simulink model "Surgical_RCM_Sim"  (R2026a)
settings: Solver=VariableStepAuto  StopTime=30.0
settings Model: Creator=shueb  LastModifiedBy=shueb

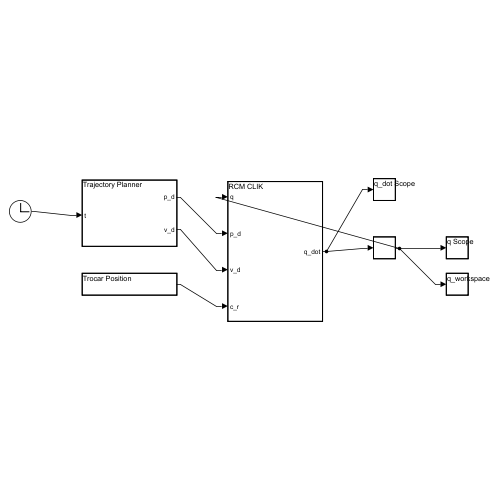
[thumbnail: Simulink's stored preview of the top-level diagram]
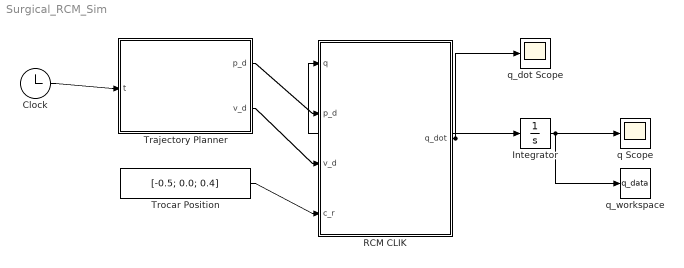
== system Surgical_RCM_Sim ==
  Clock : Clock
  Integrator : Integrator  InitialCondition=[0; 0.4085; 3.1416; 0.6128; -3.1416; 2.1203; 3.1416]
  RCM CLIK : MATLAB Function  TreatAsAtomicUnit=on
  Trajectory Planner : MATLAB Function  TreatAsAtomicUnit=on
  Trocar Position : Constant  Value=[-0.5; 0.0; 0.4]
  q Scope : Scope
  q_dot Scope : Scope
  q_workspace : ToWorkspace  VariableName=q_data  SampleTime=-1
  wires:
  Clock/1 -> Trajectory Planner/1(t)
  Trajectory Planner/1(p_d) -> RCM CLIK/2(p_d)
  Trajectory Planner/2(v_d) -> RCM CLIK/3(v_d)
  Trocar Position/1 -> RCM CLIK/4(c_r)
  Integrator/1 -> RCM CLIK/1(q), q Scope/1, q_workspace/1
  RCM CLIK/1(q_dot) -> Integrator/1, q_dot Scope/1

== matlab function Surgical_RCM_Sim/RCM CLIK ==
  data: q input; q_dot output; p_d input; v_d input; c_r input
function q_dot = rcm_clik_controller(q, p_d, v_d, c_r)
    %#codegen
    assert(isa(q, 'double'));
    assert(all(size(q) == [7, 1]));
    assert(isa(p_d, 'double'));
    assert(all(size(p_d) == [3, 1]));
    assert(isa(v_d, 'double'));
    assert(all(size(v_d) == [3, 1]));
    assert(isa(c_r, 'double'));
    assert(all(size(c_r) == [3, 1]));

    q_dot = zeros(7, 1);
    % Gains
    K_rcm = 10;
    K_tool = 5;
    
    % Forward Kinematics
    T_e = kuka_direct_kinematics(q);
    p_e = T_e(1:3, 4);
    R_e = T_e(1:3, 1:3);
    z_e = R_e(:, 3);
    
    J_e = jacobian_kuka(q);
    J_v = J_e(1:3, :);
    J_w = J_e(4:6, :);
    
    % Tool Kinematics
    L = 0.15;
    p_tool = p_e + L * z_e;
    skew_Lz = [0, -L*z_e(3), L*z_e(2);
               L*z_e(3), 0, -L*z_e(1);
               -L*z_e(2), L*z_e(1), 0];
    J_tool = J_v - skew_Lz * J_w;
    
    % RCM Kinematics
    lambda = (c_r - p_e)' * z_e;
    p_c = p_e + lambda * z_e;
    e_rcm = c_r - p_c;
    
    skew_lamz = [0, -lambda*z_e(3), lambda*z_e(2);
                 lambda*z_e(3), 0, -lambda*z_e(1);
                 -lambda*z_e(2), lambda*z_e(1), 0];
    J_pc = J_v - skew_lamz * J_w;
    
    Proj_ortho = eye(3) - z_e * z_e';
    J_rcm = Proj_ortho * J_pc;
    
    % Task-Priority CLIK
    % Task 1: RCM Constraint (highest priority)
    J_rcm_pinv = pinv(J_rcm);
    q_dot_1 = J_rcm_pinv * (K_rcm * e_rcm);
    
    % Task 2: Tool tracking (secondary priority)
    e_tool = p_d - p_tool;
    v_tool_1 = J_tool * q_dot_1;
    v_tool_req = v_d + K_tool * e_tool - v_tool_1;
    
    N_1 = eye(7) - J_rcm_pinv * J_rcm;
    J_tool_N = J_tool * N_1;
    
    % Damped Least Squares for Secondary Task to avoid singularities
    lambda_damp = 0.1;
    J_tool_N_pinv = J_tool_N' / (J_tool_N * J_tool_N' + lambda_damp^2 * eye(3));
    
    q_dot_2 = J_tool_N_pinv * v_tool_req;
    
    q_dot = q_dot_1 + q_dot_2;
end

== matlab function Surgical_RCM_Sim/Trajectory Planner ==
  data: t input; p_d output; v_d output
function [p_d, v_d] = trajectory_planner(t)
    %#codegen
    assert(isa(t, 'double'));
    assert(all(size(t) == [1, 1]));
    
    p_d = zeros(3, 1);
    v_d = zeros(3, 1);
    
    % Reachable Targets (Trocar at [-0.5; 0.0; 0.4], L = 0.15m)
    m0 = [-0.50;  0.00; 0.30]; % Starting position
    m1 = [-0.50;  0.08; 0.28]; % Target 1
    m2 = [-0.48;  0.05; 0.27]; % Target 2
    m3 = [-0.48; -0.05; 0.27]; % Target 3
    m4 = [-0.50; -0.08; 0.28]; % Target 4
    m5 = [-0.55;  0.00; 0.30]; % Target 5
    
    T_seg = 5.0; % 5 seconds per segment
    
    if t < T_seg
        p_start = m0; p_end = m1;
        tau = t;
    elseif t < 2*T_seg
        p_start = m1; p_end = m2;
        tau = t - T_seg;
    elseif t < 3*T_seg
        p_start = m2; p_end = m3;
        tau = t - 2*T_seg;
    elseif t < 4*T_seg
        p_start = m3; p_end = m4;
        tau = t - 3*T_seg;
    elseif t < 5*T_seg
        p_start = m4; p_end = m5;
        tau = t - 4*T_seg;
    else
        p_start = m5; p_end = m5;
        tau = T_seg;
    end
    
    % Cubic polynomial s(tau) from 0 to 1
    if tau <= 0
        s = 0; s_dot = 0;
    elseif tau >= T_seg
        s = 1; s_dot = 0;
    else
        s = 3*(tau/T_seg)^2 - 2*(tau/T_seg)^3;
        s_dot = (6*tau/(T_seg^2)) - (6*tau^2/(T_seg^3));
    end
    
    p_d = p_start + (p_end - p_start) * s;
    v_d = (p_end - p_start) * s_dot;
end
